simulink model "act1_simulink_sesion3"  (R2020a)
settings: Solver=ode1  StartTime=0.0  StopTime=3  FixedStep=1e-3  RelTol=1e-3
libraries: simulink_need_slupdate x6
settings Model: Creator=jaguero  LastModifiedBy=Jorjolo

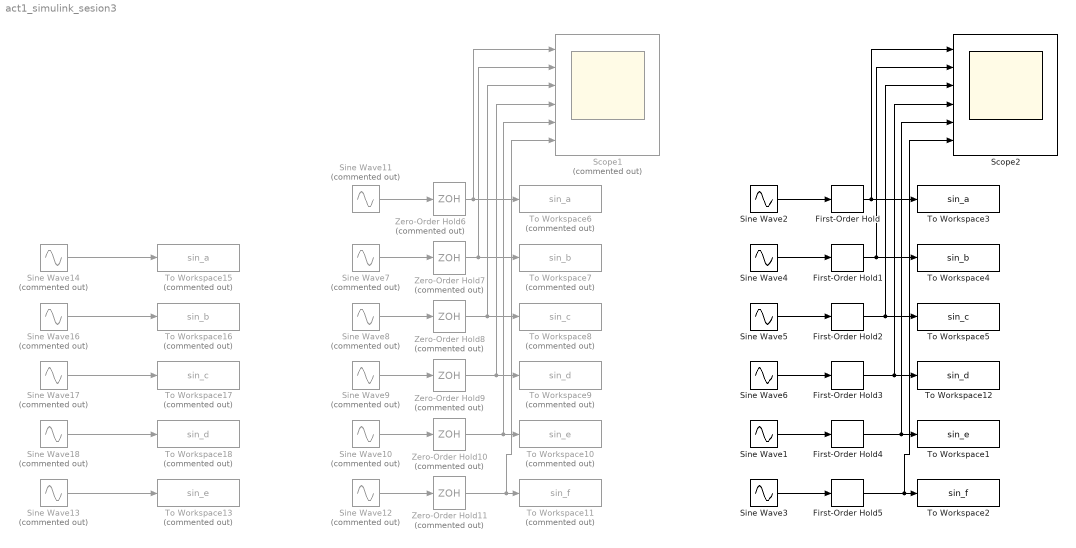
== system act1_simulink_sesion3 ==
  First-Order Hold : simulink_need_slupdate/First-Order Hold  DisableCoverage=on  Ts=0.75
      settings: SourceProductBaseCode=SL
  First-Order Hold1 : simulink_need_slupdate/First-Order Hold  DisableCoverage=on  Ts=0.5
      settings: SourceProductBaseCode=SL
  First-Order Hold2 : simulink_need_slupdate/First-Order Hold  DisableCoverage=on  Ts=0.2
      settings: SourceProductBaseCode=SL
  First-Order Hold3 : simulink_need_slupdate/First-Order Hold  DisableCoverage=on  Ts=0.1
      settings: SourceProductBaseCode=SL
  First-Order Hold4 : simulink_need_slupdate/First-Order Hold  DisableCoverage=on  Ts=0.05
      settings: SourceProductBaseCode=SL
  First-Order Hold5 : simulink_need_slupdate/First-Order Hold  DisableCoverage=on  Ts=0.01
      settings: SourceProductBaseCode=SL
  Scope1 : Scope  Commented=on  NumInputPorts=6
  Scope2 : Scope  NumInputPorts=6
  Sine Wave{1..6} (6 alike) : Sin  Frequency=2*pi  SampleTime=0
  Sine Wave{7..14,16..18} (11 alike) : Sin  Commented=on  Frequency=2*pi  SampleTime=0
  To Workspace1 : ToWorkspace  VariableName=sin_e  SaveFormat=Timeseries  SampleTime=-1
  To Workspace10 : ToWorkspace  Commented=on  VariableName=sin_e  SaveFormat=Timeseries  SampleTime=-1
  To Workspace11 : ToWorkspace  Commented=on  VariableName=sin_f  SaveFormat=Timeseries  SampleTime=-1
  To Workspace12 : ToWorkspace  VariableName=sin_d  SaveFormat=Timeseries  SampleTime=-1
  To Workspace13 : ToWorkspace  Commented=on  VariableName=sin_e  SaveFormat=Timeseries  SampleTime=0.1
  To Workspace15 : ToWorkspace  Commented=on  VariableName=sin_a  SaveFormat=Timeseries  SampleTime=0.01
  To Workspace16 : ToWorkspace  Commented=on  VariableName=sin_b  SaveFormat=Timeseries  SampleTime=0.51
  To Workspace17 : ToWorkspace  Commented=on  VariableName=sin_c  SaveFormat=Timeseries  SampleTime=0.5
  To Workspace18 : ToWorkspace  Commented=on  VariableName=sin_d  SaveFormat=Timeseries  SampleTime=0.49
  To Workspace2 : ToWorkspace  VariableName=sin_f  SaveFormat=Timeseries  SampleTime=-1
  To Workspace3 : ToWorkspace  VariableName=sin_a  SaveFormat=Timeseries  SampleTime=-1
  To Workspace4 : ToWorkspace  VariableName=sin_b  SaveFormat=Timeseries  SampleTime=-1
  To Workspace5 : ToWorkspace  VariableName=sin_c  SaveFormat=Timeseries  SampleTime=-1
  To Workspace6 : ToWorkspace  Commented=on  VariableName=sin_a  SaveFormat=Timeseries  SampleTime=-1
  To Workspace7 : ToWorkspace  Commented=on  VariableName=sin_b  SaveFormat=Timeseries  SampleTime=-1
  To Workspace8 : ToWorkspace  Commented=on  VariableName=sin_c  SaveFormat=Timeseries  SampleTime=-1
  To Workspace9 : ToWorkspace  Commented=on  VariableName=sin_d  SaveFormat=Timeseries  SampleTime=-1
  Zero-Order Hold10 : ZeroOrderHold  Commented=on  SampleTime=0.05
  Zero-Order Hold11 : ZeroOrderHold  Commented=on  SampleTime=0.01
  Zero-Order Hold6 : ZeroOrderHold  Commented=on  SampleTime=0.75
  Zero-Order Hold7 : ZeroOrderHold  Commented=on  SampleTime=0.5
  Zero-Order Hold8 : ZeroOrderHold  Commented=on  SampleTime=0.2
  Zero-Order Hold9 : ZeroOrderHold  Commented=on  SampleTime=0.1
  wires:
  Sine Wave12/1 -> Zero-Order Hold11/1
  Zero-Order Hold11/1 -> Scope1/6, To Workspace11/1
  Sine Wave9/1 -> Zero-Order Hold9/1
  Zero-Order Hold7/1 -> Scope1/2, To Workspace7/1
  Zero-Order Hold8/1 -> Scope1/3, To Workspace8/1
  Zero-Order Hold6/1 -> Scope1/1, To Workspace6/1
  Sine Wave8/1 -> Zero-Order Hold8/1
  Sine Wave10/1 -> Zero-Order Hold10/1
  Zero-Order Hold10/1 -> Scope1/5, To Workspace10/1
  Sine Wave7/1 -> Zero-Order Hold7/1
  Sine Wave11/1 -> Zero-Order Hold6/1
  Zero-Order Hold9/1 -> Scope1/4, To Workspace9/1
  First-Order Hold3/1 -> Scope2/4, To Workspace12/1
  Sine Wave1/1 -> First-Order Hold4/1
  First-Order Hold4/1 -> Scope2/5, To Workspace1/1
  Sine Wave4/1 -> First-Order Hold1/1
  Sine Wave5/1 -> First-Order Hold2/1
  Sine Wave2/1 -> First-Order Hold/1
  First-Order Hold2/1 -> Scope2/3, To Workspace5/1
  Sine Wave6/1 -> First-Order Hold3/1
  First-Order Hold5/1 -> Scope2/6, To Workspace2/1
  Sine Wave3/1 -> First-Order Hold5/1
  First-Order Hold1/1 -> Scope2/2, To Workspace4/1
  First-Order Hold/1 -> Scope2/1, To Workspace3/1
  Sine Wave16/1 -> To Workspace16/1
  Sine Wave17/1 -> To Workspace17/1
  Sine Wave14/1 -> To Workspace15/1
  Sine Wave18/1 -> To Workspace18/1
  Sine Wave13/1 -> To Workspace13/1
